simulink model "CraneModel_Final"  (R2022b)
settings: Solver=FixedStepAuto  StartTime=0.0  StopTime=15  FixedStep=0.002  RelTol=1e-3
values from neighbouring files (symbols this model uses):
  fHeightKingActLower = 0.161    [craneParameters.m]
  fHeightKingActUpper = 0.130    (= 0.13)    [craneParameters.m]
  fHeightKingSlew = 0.623    [craneParameters.m]
  fHeightKnuckleActLower = 0.160    (= 0.16)    [craneParameters.m]
  fHeightKnuckleActUpper = 0.182    [craneParameters.m]
  fHeightPlatform = 1.402    [craneParameters.m]
  fHeightPlatformKing = 0.09    [craneParameters.m]
  fHeightSlewTop = 0.711    [craneParameters.m]
  fHeightToSheave1 = 0.060    (= 0.06)    [craneParameters.m]
  fHeightToSheave2 = 0.095    [craneParameters.m]
  fHeightToSheave3 = 0.198    [craneParameters.m]
  fHeightToSheave4 = 1.158    [craneParameters.m]
  fHeightToWinch = 0.0895    [craneParameters.m]
  fLengthKingActLower = 0.154    [craneParameters.m]
  fLengthKingActUpper = 0.600    (= 0.6)    [craneParameters.m]
  fLengthKnuckleActLower = 0.750    (= 0.75)    [craneParameters.m]
  fLengthKnuckleActUpper = 0.027    [craneParameters.m]
  fLengthMainArm = 1.5    [craneParameters.m]
  fLengthPlatform = 1.30    (= 1.3)    [craneParameters.m]
  fLengthToSheave1 = 0.235    [craneParameters.m]
  fLengthToSheave2 = 1.520    (= 1.52)    [craneParameters.m]
  fLengthToSheave3 = 0.168    [craneParameters.m]
  fLengthToSheave4 = 0    [craneParameters.m]
  fLengthToWinch = 0.22    [craneParameters.m]
  fMinLengthActuatorKnuckle = 0.633    [craneParameters.m]
  fMinLengthActuatorMain = 0.691    [craneParameters.m]
  massActuatorBottomMain = 14    [craneParameters.m]
  massActuatorBottomRod = 3    [craneParameters.m]
  massActuatorTopMain = 14    [craneParameters.m]
  massKingBottom = 92.2    [craneParameters.m]
  massKingMountingPlate = 58.2    [craneParameters.m]
  massKingTop = 63.6    [craneParameters.m]
  massKnuckleArm = 8.7    [craneParameters.m]
  massMainArm = 12.5    [craneParameters.m]
  massPayload = 13.5    [craneParameters.m]
  massTestRigBase = 924    [craneParameters.m]
  massTestRigPlatform = 268    [craneParameters.m]
  massWinch = 4.8    [craneParameters.m]
  massWinchDrum = 2.3    [craneParameters.m]
  sheavePitchRadius = sheavePitchDiameter/2    (= 0.034)    [craneParameters.m]
  winchGearRatio = 32    [craneParameters.m]    (also in winchCalculations.m)
undefined symbols (not defined in the file or in its folder): X, Y, Z
libraries: sm_lib x138, nesl_utility x20, vrlib x1, sldrtlib x1
(part 1 of 4)
settings Model: Creator=krgar  LastModifiedBy=krgar
settings ConfigComp: PLC_TargetIDE=plcopen  PLC_MultiTBSigbuilderTimeRange=off  PLC_FoldFBCallOutputVar=off  PLC_InlineEnumCastFunction=off

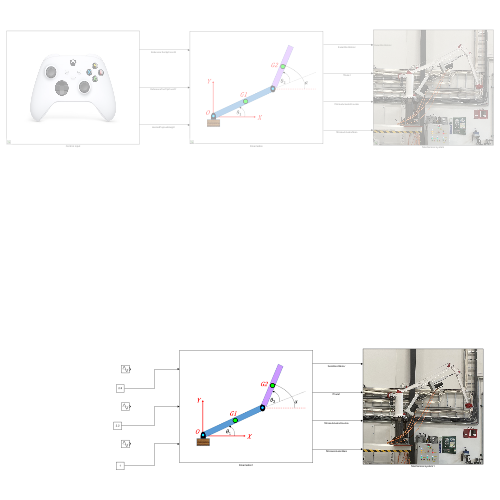
[thumbnail: Simulink's stored preview of the top-level diagram]
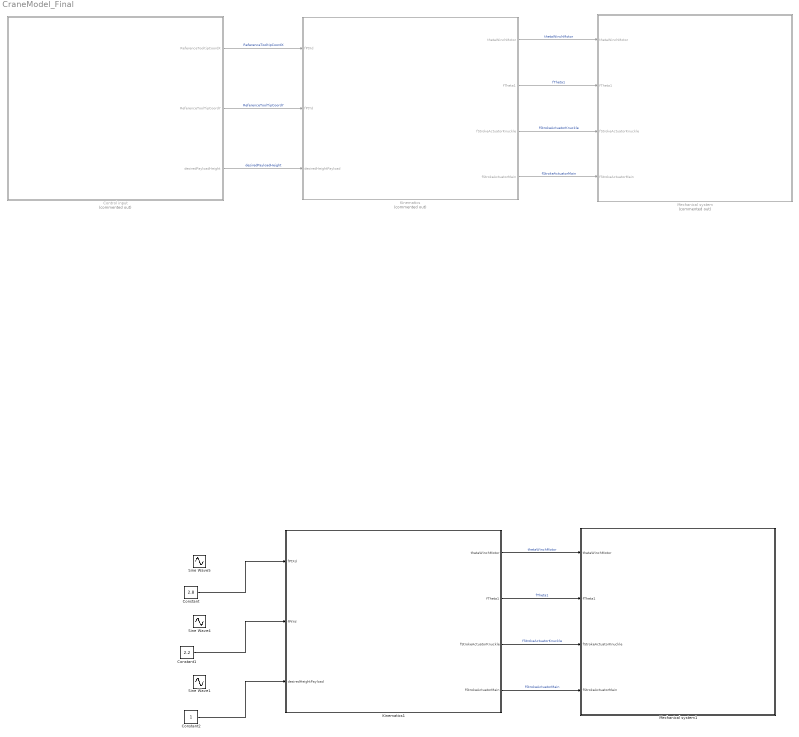
== system CraneModel_Final ==
  Constant : Constant  Value=2.8
  Constant1 : Constant  Value=2.2
  Constant2 : Constant
  Control input : Subsystem  Commented=on
      mask Display: image('.\Mask\Xbox.jpg'); % Use "Edit Image" on toolstrip to change.
  Kinematics : Subsystem  Commented=on
      mask Display: image('.\Mask\Kinematics.png'); % Use "Edit Image" on toolstrip to change.
  Kinematics1 : Subsystem
      mask Display: image('.\Mask\Kinematics.png'); % Use "Edit Image" on toolstrip to change.
  Mechanical system : Subsystem  Commented=on
      mask Display: image('.\Mask\Crane.jpg'); % Use "Edit Image" on toolstrip to change.
  Mechanical system1 : Subsystem
      mask Display: image('.\Mask\Crane.jpg'); % Use "Edit Image" on toolstrip to change.
  Sine Wave1 : Sin  Amplitude=0.5  Bias=0.5  SampleTime=0
  Sine Wave4 : Sin  Amplitude=0.1  Bias=2.2  SampleTime=0
  Sine Wave5 : Sin  Amplitude=0.1  Bias=3.3  SampleTime=0
  wires:
  Kinematics/1(thetaWinchMotor) -> Mechanical system/1(thetaWinchMotor)  "thetaWinchMotor"
  Kinematics/2(fTheta1) -> Mechanical system/2(fTheta1)  "fTheta1"
  Kinematics/3(fStrokeActuatorKnuckle) -> Mechanical system/3(fStrokeActuatorKnuckle)  "fStrokeActuatorKnuckle"
  Kinematics/4(fStrokeActuatorMain) -> Mechanical system/4(fStrokeActuatorMain)  "fStrokeActuatorMain"
  Control input/1(ReferenceTooltipCoordX) -> Kinematics/1(fPtXd)  "ReferenceTooltipCoordX"
  Control input/2(ReferenceToolTipCoordY) -> Kinematics/2(fPtYd)  "ReferenceToolTipCoordY"
  Control input/3(desiredPayloadHeight) -> Kinematics/3(desiredHeightPayload)  "desiredPayloadHeight"
  Kinematics1/4(fStrokeActuatorMain) -> Mechanical system1/4(fStrokeActuatorMain)  "fStrokeActuatorMain"
  Kinematics1/3(fStrokeActuatorKnuckle) -> Mechanical system1/3(fStrokeActuatorKnuckle)  "fStrokeActuatorKnuckle"
  Kinematics1/2(fTheta1) -> Mechanical system1/2(fTheta1)  "fTheta1"
  Kinematics1/1(thetaWinchMotor) -> Mechanical system1/1(thetaWinchMotor)  "thetaWinchMotor"
  Constant2/1 -> Kinematics1/3(desiredHeightPayload)
  Constant1/1 -> Kinematics1/2(fPtYd)
  Constant/1 -> Kinematics1/1(fPtXd)

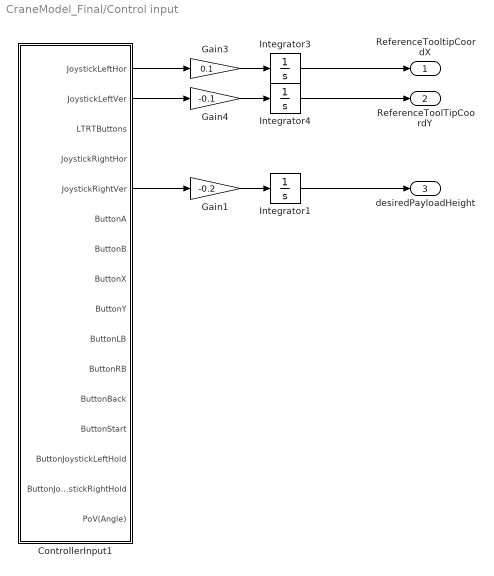
== system CraneModel_Final/Control input ==
  ControllerInput1 : Subsystem
  Gain1 : Gain  Gain=-0.2
  Gain3 : Gain  Gain=0.1
  Gain4 : Gain  Gain=-0.1
  Integrator1 : Integrator
  Integrator3 : Integrator  InitialCondition=3.2
  Integrator4 : Integrator  InitialCondition=2.5
  ReferenceTooltipCoordX : Outport
  ReferenceToolTipCoordY : Outport  Port=2
  desiredPayloadHeight : Outport  Port=3
  wires:
  ControllerInput1/1(JoystickLeftHor) -> Gain3/1
  ControllerInput1/2(JoystickLeftVer) -> Gain4/1
  Integrator3/1 -> ReferenceTooltipCoordX/1
  ControllerInput1/5(JoystickRightVer) -> Gain1/1
  Gain3/1 -> Integrator3/1
  Gain4/1 -> Integrator4/1
  Gain1/1 -> Integrator1/1
  Integrator4/1 -> ReferenceToolTipCoordY/1
  Integrator1/1 -> desiredPayloadHeight/1

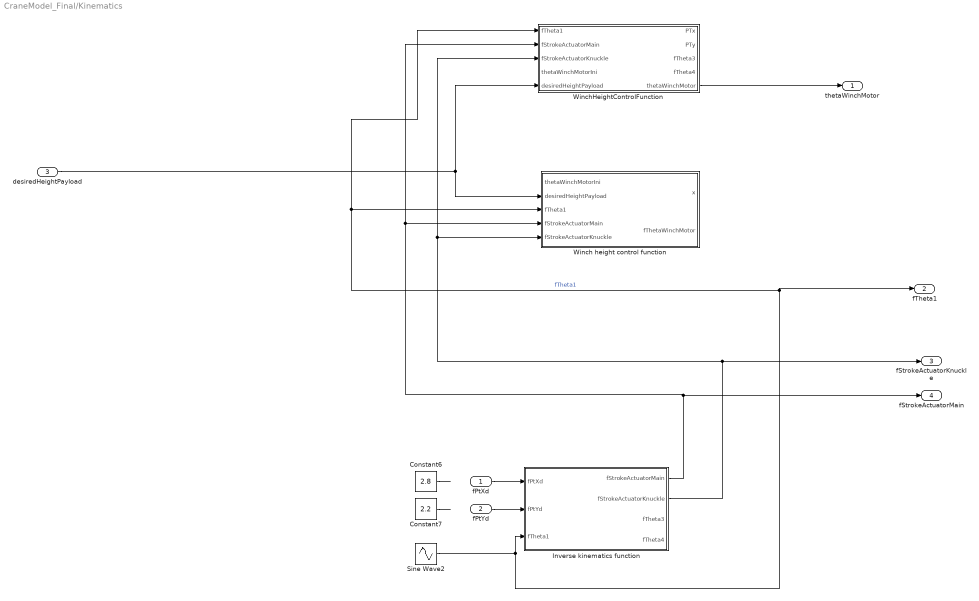
== system CraneModel_Final/Kinematics ==
  fPtXd : Inport
  fPtYd : Inport  Port=2
  desiredHeightPayload : Inport  Port=3
  Constant6 : Constant  Value=2.8
  Constant7 : Constant  Value=2.2
  Inverse kinematics function : MATLAB Function  TreatAsAtomicUnit=on
  Sine Wave2 : Sin  Amplitude=0.05  SampleTime=0
  Winch height control function : Subsystem  TreatAsAtomicUnit=on
  WinchHeightControlFunction : MATLAB Function  TreatAsAtomicUnit=on
  thetaWinchMotor : Outport
  fTheta1 : Outport  Port=2
  fStrokeActuatorKnuckle : Outport  Port=3
  fStrokeActuatorMain : Outport  Port=4
  wires:
  Inverse kinematics function/2(fStrokeActuatorKnuckle) -> fStrokeActuatorKnuckle/1, WinchHeightControlFunction/3(fStrokeActuatorKnuckle), Winch height control function/5(fStrokeActuatorKnuckle)
  Inverse kinematics function/1(fStrokeActuatorMain) -> fStrokeActuatorMain/1, WinchHeightControlFunction/2(fStrokeActuatorMain), Winch height control function/4(fStrokeActuatorMain)
  Sine Wave2/1 -> Inverse kinematics function/3(fTheta1), WinchHeightControlFunction/1(fTheta1), Winch height control function/3(fTheta1), fTheta1/1  "fTheta1"
  desiredHeightPayload/1 -> Winch height control function/2(desiredHeightPayload), WinchHeightControlFunction/5(desiredHeightPayload)
  Constant7/1 -> ?
  fPtYd/1 -> Inverse kinematics function/2(fPtYd)
  Constant6/1 -> ?
  fPtXd/1 -> Inverse kinematics function/1(fPtXd)
  WinchHeightControlFunction/5(thetaWinchMotor) -> thetaWinchMotor/1

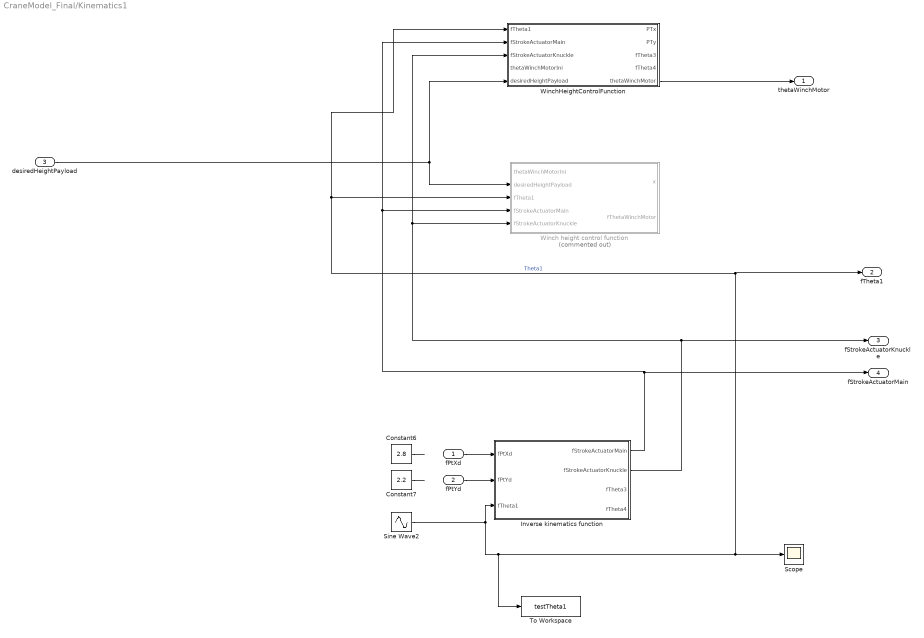
== system CraneModel_Final/Kinematics1 ==
  fPtXd : Inport
  fPtYd : Inport  Port=2
  desiredHeightPayload : Inport  Port=3
  Constant6 : Constant  Value=2.8
  Constant7 : Constant  Value=2.2
  Inverse kinematics function : MATLAB Function  TreatAsAtomicUnit=on
  Scope : Scope
  Sine Wave2 : Sin  Amplitude=0.05  SampleTime=0
  To Workspace : ToWorkspace  VariableName=testTheta1  SaveFormat=Timeseries  SampleTime=-1
      settings: Save2DSignal=2-D array (concatenate along first dimension)
  Winch height control function : Subsystem  Commented=on  TreatAsAtomicUnit=on
  WinchHeightControlFunction : MATLAB Function  TreatAsAtomicUnit=on
  thetaWinchMotor : Outport
  fTheta1 : Outport  Port=2
  fStrokeActuatorKnuckle : Outport  Port=3
  fStrokeActuatorMain : Outport  Port=4
  wires:
  Inverse kinematics function/2(fStrokeActuatorKnuckle) -> fStrokeActuatorKnuckle/1, WinchHeightControlFunction/3(fStrokeActuatorKnuckle), Winch height control function/5(fStrokeActuatorKnuckle)
  Inverse kinematics function/1(fStrokeActuatorMain) -> fStrokeActuatorMain/1, WinchHeightControlFunction/2(fStrokeActuatorMain), Winch height control function/4(fStrokeActuatorMain)
  Sine Wave2/1 -> Inverse kinematics function/3(fTheta1), To Workspace/1, Scope/1, WinchHeightControlFunction/1(fTheta1), Winch height control function/3(fTheta1), fTheta1/1  "Theta1"
  desiredHeightPayload/1 -> Winch height control function/2(desiredHeightPayload), WinchHeightControlFunction/5(desiredHeightPayload)
  Constant7/1 -> ?
  fPtYd/1 -> Inverse kinematics function/2(fPtYd)
  Constant6/1 -> ?
  fPtXd/1 -> Inverse kinematics function/1(fPtXd)
  WinchHeightControlFunction/5(thetaWinchMotor) -> thetaWinchMotor/1
